simulink model "HDLRxSeparated"  (R2024a)
settings: Solver=FixedStepDiscrete  StartTime=0.0  StopTime=stopTime  RelTol=1e-3
values from neighbouring files (symbols this model uses):
  msgQtty = length(msgIn)    [testRx.m]
undefined symbols (not defined in the file or in its folder): CONST
libraries: HDL_ieee_8021513 x4, hdlsllib x2, dspsrcs4 x2
settings Model: DataTypeOverride=Off  SimulationMode=accelerator  Creator=cotti  LastModifiedBy=cotti
settings OptimizationCC: BlockReduction=off  ConditionallyExecuteInputs=off  DefaultParameterBehavior=Inlined  InheritOutputTypeSmallerThanSingle=on
settings DebuggingCC: AlgebraicLoopMsg=error  ArtificialAlgebraicLoopMsg=error  SingleTaskRateTransMsg=error  UnconnectedInputMsg=warning  UnconnectedOutputMsg=warning  UnconnectedLineMsg=warning
settings HardwareCC: ProdBitPerPointer=32  ProdBitPerSizeT=32  ProdBitPerPtrDiffT=32  ProdLargestAtomicFloat=None  ProdIntDivRoundTo=Undefined  ProdEndianess=Unspecified  ProdWordSize=32  ProdHWDeviceType=ASIC/FPGA->ASIC/FPGA  TargetBitPerLong=64  TargetBitPerPointer=64  TargetBitPerSizeT=64  TargetBitPerPtrDiffT=64  TargetLongLongMode=on  TargetIntDivRoundTo=Zero  TargetEndianess=LittleEndian  TargetWordSize=64  TargetHWDeviceType=Custom Processor->MATLAB Host Computer  ProdEqTarget=off

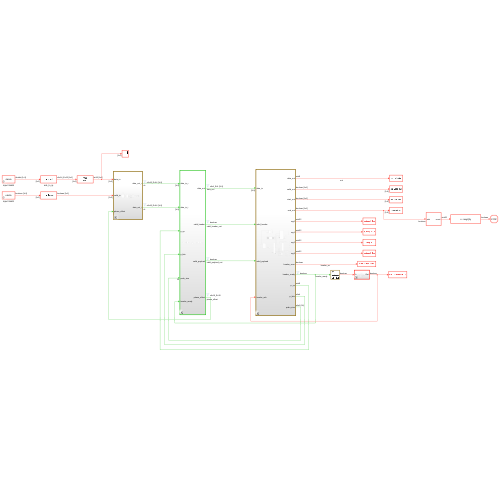
[thumbnail: Simulink's stored preview of the top-level diagram]
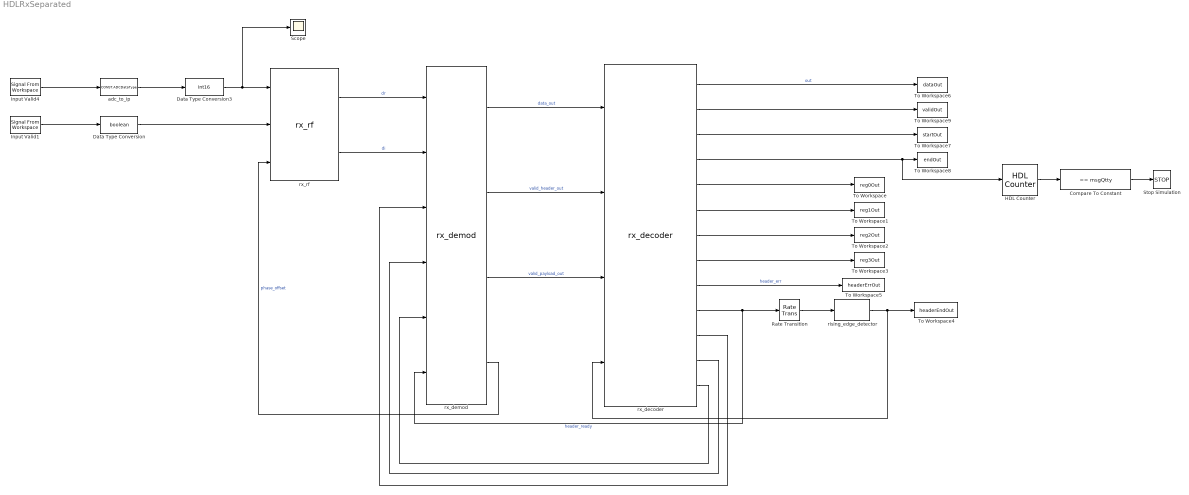
== system HDLRxSeparated ==
  Compare To Constant : hdlsllib/Logic and Bit Operations/Compare To Constant  relop===  const=msgQtty  OutDataTypeStr=boolean
  Data Type Conversion : DataTypeConversion  OutDataTypeStr=boolean  SaturateOnIntegerOverflow=off  RndMeth=Floor
  Data Type Conversion3 : DataTypeConversion  OutDataTypeStr=int16  ConvertRealWorld=Stored Integer (SI)  SaturateOnIntegerOverflow=off  RndMeth=Floor
  HDL Counter : hdlsllib/Sources/HDL Counter  CountType=Free running  CountInit=0  CountStep=1  CountMax=25  CountFromType=Initial value  CountFrom=0  CountResetPort=off  CountLoadPort=off  CountEnbPort=on  CountDirPort=off  CountHitOutputPort=off  CountDataType=Unsigned  CountWordLen=32  CountFracLen=0  CountSampTime=1
  Input Valid1 : dspsrcs4/Signal From Workspace  X=validIn  Ts=1/CONST.fADC  nsamps=1  OutputAfterFinalValue=Setting to zero  ignoreOrWarnInputAndFrameLengths=off  OutputFrames=off
  Input Valid4 : dspsrcs4/Signal From Workspace  X=dataIn  Ts=1/CONST.fADC  nsamps=1  OutputAfterFinalValue=Setting to zero  ignoreOrWarnInputAndFrameLengths=off  OutputFrames=off
  Rate Transition : RateTransition  OutPortSampleTime=1/CONST.fs
  Scope : Scope
  Stop Simulation : Stop
  To Workspace : ToWorkspace  VariableName=reg0Out  SampleTime=1/CONST.fs
      settings: Save2DSignal=2-D array (concatenate along first dimension)
  To Workspace1 : ToWorkspace  VariableName=reg1Out  SampleTime=1/CONST.fs
      settings: Save2DSignal=2-D array (concatenate along first dimension)
  To Workspace2 : ToWorkspace  VariableName=reg2Out  SampleTime=1/CONST.fs
      settings: Save2DSignal=2-D array (concatenate along first dimension)
  To Workspace3 : ToWorkspace  VariableName=reg3Out  SampleTime=1/CONST.fs
      settings: Save2DSignal=2-D array (concatenate along first dimension)
  To Workspace4 : ToWorkspace  VariableName=headerEndOut  SampleTime=1/CONST.fs
      settings: Save2DSignal=2-D array (concatenate along first dimension)
  To Workspace5 : ToWorkspace  VariableName=headerErrOut  SampleTime=1/CONST.fs
      settings: Save2DSignal=2-D array (concatenate along first dimension)
  To Workspace6 : ToWorkspace  VariableName=dataOut  SampleTime=1/CONST.fs
      settings: Save2DSignal=2-D array (concatenate along first dimension)
  To Workspace7 : ToWorkspace  VariableName=startOut  SampleTime=1/CONST.fs
      settings: Save2DSignal=2-D array (concatenate along first dimension)
  To Workspace8 : ToWorkspace  VariableName=endOut  SampleTime=1/CONST.fs
      settings: Save2DSignal=2-D array (concatenate along first dimension)
  To Workspace9 : ToWorkspace  VariableName=validOut  SampleTime=1/CONST.fs
      settings: Save2DSignal=2-D array (concatenate along first dimension)
  adc_to_ip : DataTypeConversion  OutDataTypeStr=CONST.ADCDataType  SaturateOnIntegerOverflow=off  RndMeth=Floor
  rising_edge_detector : HDL_ieee_8021513/rising_edge_detector  SystemSampleTime=-1  VariantActivationTime=update diagram  AllowFlexibleInterface=on  Latency=0  AutoFrameSizeCalculation=off
      settings: SourceProductName=HDL IEEE 8021513
  rx_decoder : HDL_ieee_8021513/rx_decoder  SystemSampleTime=-1  VariantActivationTime=update diagram  AllowFlexibleInterface=on  Latency=0  AutoFrameSizeCalculation=off
      settings: SourceProductName=HDL IEEE 8021513
  rx_demod : HDL_ieee_8021513/rx_demod  SystemSampleTime=-1  VariantActivationTime=update diagram  AllowFlexibleInterface=on  Latency=0  AutoFrameSizeCalculation=off
      settings: SourceProductName=HDL IEEE 8021513
  rx_rf : HDL_ieee_8021513/rx_rf  SystemSampleTime=-1  VariantActivationTime=update diagram  AllowFlexibleInterface=on  Latency=0  AutoFrameSizeCalculation=off
      settings: SourceProductName=HDL IEEE 8021513
  wires:
  rx_rf/1 -> rx_demod/1  "dr"
  rx_rf/2 -> rx_demod/2  "di"
  rx_demod/4 -> rx_rf/3  "phase_offset"
  rx_demod/1 -> rx_decoder/1  "data_out"
  rx_demod/2 -> rx_decoder/2  "valid_header_out"
  rx_demod/3 -> rx_decoder/3  "valid_payload_out"
  Input Valid4/1 -> adc_to_ip/1
  adc_to_ip/1 -> Data Type Conversion3/1
  Input Valid1/1 -> Data Type Conversion/1
  Data Type Conversion/1 -> rx_rf/2
  rx_decoder/6 -> To Workspace1/1
  rx_decoder/7 -> To Workspace2/1
  rx_decoder/2 -> To Workspace9/1
  rx_decoder/8 -> To Workspace3/1
  rx_decoder/1 -> To Workspace6/1  "out"
  rx_decoder/3 -> To Workspace7/1
  Compare To Constant/1 -> Stop Simulation/1
  rx_decoder/10 -> rx_demod/6, Rate Transition/1  "header_ready"
  HDL Counter/1 -> Compare To Constant/1
  rx_decoder/9 -> To Workspace5/1  "header_err"
  rx_decoder/5 -> To Workspace/1
  rx_decoder/4 -> HDL Counter/1, To Workspace8/1
  rising_edge_detector/1 -> rx_decoder/4, To Workspace4/1
  rx_decoder/13 -> rx_demod/5
  rx_decoder/12 -> rx_demod/4
  rx_decoder/11 -> rx_demod/3
  Rate Transition/1 -> rising_edge_detector/1
  Data Type Conversion3/1 -> Scope/1, rx_rf/1
